simulink model "BenchmarkModel_Phasor"  (R2020a)
settings: Solver=VariableStepAuto  StartTime=0.0  StopTime=24*3600  RelTol=1e-3
undefined symbols (not defined in the file): A, a, Ac, B, Bc, C, Cc, Dc, Dd, find_system, Fnom, gcbh, I21_init_imag, I21_init_real, Ibase1, Ibase2, Iw1A_init_mag, Iw1A_init_pha, Iw1B_init_mag, Iw1B_init_pha, Iw1C_init_mag, Iw1C_init_pha, Iw2A_init_mag, Iw2A_init_pha, Iw2B_init_mag, Iw2B_init_pha, Iw2C_init_mag, Iw2C_init_pha, j, kr, ks, Nmax, Pnom, psi, sps_rtmsupport, V2G, Vnom1, Vnom2, w, Z1pu, Z2pu, Ztpu
libraries: powerlib x58, simulink x7, powerlib_meascontrol x7
(part 2 of 3)

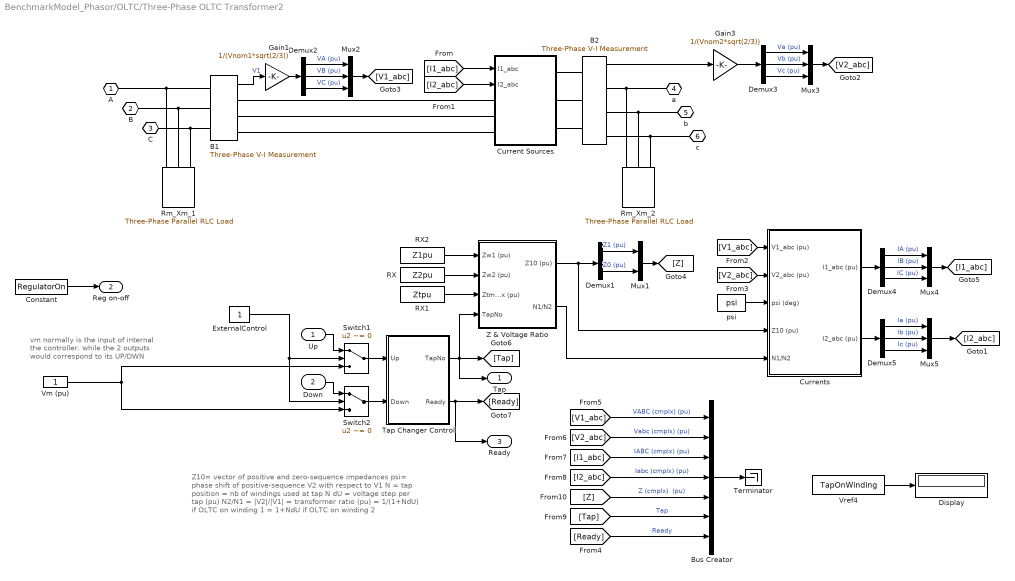
== system BenchmarkModel_Phasor/OLTC/Three-Phase OLTC Transformer2 ==
  note: vm normally is the input of
      | internal the controller.
      | while the 2 outputs would
      | correspond to its UP/DWN
  note: Z10= vector of positive and zero-sequence impedances
      | psi= phase shift of positive-sequence V2 with respect to V1
      | N =  tap position = nb of windings used at tap N
      | dU = voltage step  per tap (pu)
      | N2/N1 =  |V2|/|V1| = transformer ratio  (pu)
      |             = 1/(1+NdU)  if OLTC on winding 1
      |             = 1+NdU        if OLTC on winding 2
  Up : Inport
  Down : Inport  Port=2
  " Currents " : Subsystem
  "B1 " : powerlib/Measurements/Three-Phase V-I Measurement  VoltageMeasurement=phase-to-ground  SetLabelV=off  LabelV=Vabc_B21  Vpu=off  VpuLL=off  CurrentMeasurement=no  SetLabelI=off  LabelI=Iabc_B21  Ipu=off  Pbase=10e6  Vbase=Us  OutputType=Complex  PhasorSimulation=on  PSBequivalent=0
  B2 : powerlib/Measurements/Three-Phase V-I Measurement  VoltageMeasurement=phase-to-ground  SetLabelV=off  LabelV=Vabc_B21  Vpu=off  VpuLL=off  CurrentMeasurement=no  SetLabelI=off  LabelI=Iabc_B21  Ipu=off  Pbase=10e6  Vbase=Us  OutputType=Complex  PhasorSimulation=on  PSBequivalent=0
  Bus Creator : BusCreator  Inputs=7
  Constant : Constant  Value=RegulatorOn
  Current Sources : Subsystem
  Demux1 : Demux  Outputs=2
      settings: DisplayOption=none
  Demux{2..5} (4 alike) : Demux  Outputs=3
      settings: DisplayOption=none
  Display : Display
  ExternalControl : Constant
  Gain1 : Gain  Gain=1/(Vnom1*sqrt(2/3))  SaturateOnIntegerOverflow=on  OutDataTypeStr=Inherit: Same as input  ParamDataTypeStr=Inherit: Same as input
  Gain3 : Gain  Gain=1/(Vnom2*sqrt(2/3))  SaturateOnIntegerOverflow=on  OutDataTypeStr=Inherit: Same as input  ParamDataTypeStr=Inherit: Same as input
  Mux1 : Mux  Inputs=2
  Mux{2..5} (4 alike) : Mux  Inputs=3
  RX : Constant  Value=Z2pu
  RX1 : Constant  Value=Ztpu
  RX2 : Constant  Value=Z1pu
  Rm_Xm_1 : powerlib/Elements/Three-Phase Parallel RLC Load  LConnTagsString=A|B|C  Configuration=Y (grounded)  NominalVoltage=Vnom1  Vabc=[1e3 1e3 1e3]  Vabcp=[1e3 1e3 1e3]  NominalFrequency=Fnom  UnbalancedPower=off  ActivePower=Pnom/RmXm(1)/2  InductivePower=Pnom/RmXm(2)/2  CapacitivePower=0  Pabc=[10e3 9e3 11e3]  QLabc=[100 90 110]  QCabc=[100 90 110]  Pabcp=[10e3 9e3 11e3]  QLabcp=[100 90 110]  QCabcp=[100 90 110]  Measurements=None  LoadType=constant Z
  Rm_Xm_2 : powerlib/Elements/Three-Phase Parallel RLC Load  LConnTagsString=A|B|C  Configuration=Y (grounded)  NominalVoltage=Vnom2  Vabc=[1e3 1e3 1e3]  Vabcp=[1e3 1e3 1e3]  NominalFrequency=Fnom  UnbalancedPower=off  ActivePower=Pnom/RmXm(1)/2  InductivePower=Pnom/RmXm(2)/2  CapacitivePower=0  Pabc=[10e3 9e3 11e3]  QLabc=[100 90 110]  QCabc=[100 90 110]  Pabcp=[10e3 9e3 11e3]  QLabcp=[100 90 110]  QCabcp=[100 90 110]  Measurements=None  LoadType=constant Z
  Switch1 : Switch  Criteria=u2 ~= 0
  Switch2 : Switch  Criteria=u2 ~= 0
  Tap Changer Control : Subsystem  mask(Tap Changer Control){MinMaxTap=TapMinMax, InitialPosition=InitialTap, MecDelay=TapSelectionTime}
      mask prompts: MinMaxTap "Minimum and maximum tap number [ Min  Max ] :"; InitialPosition "Initial tap position"; MecDelay "Mechanical delay time"
      mask init:
      | if MecDelay<=0,
      | 	MecDelay=1/60;
      | end
  Terminator : Terminator
  Vm (pu) : Constant
  Vref4 : Constant  Value=TapOnWinding
  Z & Voltage Ratio : Subsystem
  psi : Constant  Value=psi
  A : PMIOPort  Tag=PMCPort  Side=Left
  B : PMIOPort  Tag=PMCPort  Port=2  Side=Left
  C : PMIOPort  Tag=PMCPort  Port=3  Side=Left
  a : PMIOPort  Tag=PMCPort  Port=4  Side=Right
  b : PMIOPort  Tag=PMCPort  Port=5  Side=Right
  c : PMIOPort  Tag=PMCPort  Port=6  Side=Right
  Tap : Outport
  Reg on-off : Outport  Port=2
  Ready : Outport  Port=3
  wires:
  [Ready] -> Bus Creator/7  "Ready"
  Constant/1 -> Reg on-off/1
  Switch2/1 -> Tap Changer Control/2("Down ")
  ExternalControl/1 -> Switch2/2, Switch1/2
  Down/1 -> Switch2/1
  Up/1 -> Switch1/1
  Switch1/1 -> Tap Changer Control/1("Up ")
  Vm (pu)/1 -> Switch2/3, Switch1/3
  Tap Changer Control/2(Ready) -> Ready/1, [Ready]
  Tap Changer Control/1(TapNo) -> Tap/1, Z & Voltage Ratio/4(TapNo), [Tap]
  "B1 "/1 -> Gain1/1  "V1"
  RX/1 -> Z & Voltage Ratio/2(Zw2 (pu))
  RX1/1 -> Z & Voltage Ratio/3(Ztmax (pu))
  Z & Voltage Ratio/1("Z10 (pu) ") -> Demux1/1, " Currents "/4(Z10 (pu))
  RX2/1 -> Z & Voltage Ratio/1(Zw1 (pu))
  Z & Voltage Ratio/2(N1/N2) -> " Currents "/5(N1/N2)
  [I1_abc] -> Current Sources/1(I1_abc)
  [I2_abc] -> Current Sources/2(I2_abc)
  B2/1 -> Gain3/1
  Gain3/1 -> Demux3/1
  Gain1/1 -> Demux2/1
  [V1_abc] -> " Currents "/1(V1_abc (pu))
  [V2_abc] -> " Currents "/2(V2_abc (pu))
  psi/1 -> " Currents "/3(psi (deg))
  [V2_abc] -> Bus Creator/2  "Vabc (cmplx) (pu)"
  Bus Creator/1 -> Terminator/1
  [I1_abc] -> Bus Creator/3  "IABC (cmplx) (pu)"
  [I2_abc] -> Bus Creator/4  "Iabc (cmplx) (pu)"
  [Tap] -> Bus Creator/6  "Tap"
  Demux1/1 -> Mux1/1  "Z1 (pu)"
  Demux1/2 -> Mux1/2  "Z0 (pu)"
  Mux1/1 -> [Z]
  [Z] -> Bus Creator/5  "Z (cmplx)  (pu)"
  Demux2/1 -> Mux2/1  "VA (pu)"
  Demux2/2 -> Mux2/2  "VB (pu)"
  Demux2/3 -> Mux2/3  "VC (pu)"
  Mux2/1 -> [V1_abc]
  [V1_abc] -> Bus Creator/1  "VABC (cmplx) (pu)"
  Demux3/1 -> Mux3/1  "Va (pu)"
  Demux3/2 -> Mux3/2  "Vb (pu)"
  Demux3/3 -> Mux3/3  "Vc (pu)"
  Mux3/1 -> [V2_abc]
  Demux4/1 -> Mux4/1  "IA (pu)"
  Demux4/2 -> Mux4/2  "IB (pu)"
  Demux4/3 -> Mux4/3  "IC (pu)"
  Mux4/1 -> [I1_abc]
  " Currents "/1(I1_abc (pu)) -> Demux4/1
  Demux5/1 -> Mux5/1  "Ia (pu)"
  Demux5/2 -> Mux5/2  "Ib (pu)"
  Demux5/3 -> Mux5/3  "Ic (pu)"
  Mux5/1 -> [I2_abc]
  " Currents "/2("I2_abc (pu) ") -> Demux5/1
  Vref4/1 -> Display/1
  connections:
  Current Sources/RConn3 -- B2/LConn3
  Current Sources/RConn2 -- B2/LConn2
  Current Sources/RConn1 -- B2/LConn1
  "B1 "/RConn3 -- Current Sources/LConn3
  "B1 "/RConn2 -- Current Sources/LConn2
  Current Sources/LConn1 -- "B1 "/RConn1
  A/RConn1 -- "B1 "/LConn1 -- Rm_Xm_1/LConn1
  B/RConn1 -- "B1 "/LConn2 -- Rm_Xm_1/LConn2
  C/RConn1 -- "B1 "/LConn3 -- Rm_Xm_1/LConn3
  c/RConn1 -- B2/RConn3 -- Rm_Xm_2/LConn3
  b/RConn1 -- B2/RConn2 -- Rm_Xm_2/LConn2
  a/RConn1 -- B2/RConn1 -- Rm_Xm_2/LConn1

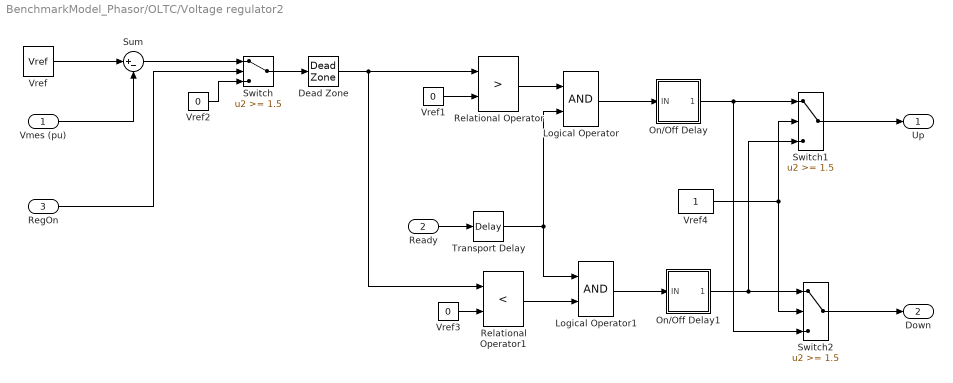
== system BenchmarkModel_Phasor/OLTC/Voltage regulator2 ==
  Vmes (pu) : Inport
  Ready : Inport  Port=2
  RegOn : Inport  Port=3
  Dead Zone : DeadZone  LowerValue=-DeadBand/2  UpperValue=+DeadBand/2  SaturateOnIntegerOverflow=on
  Logical Operator : Logic  AllPortsSameDT=off
  Logical Operator1 : Logic  AllPortsSameDT=off
  On/Off Delay : Subsystem  DialogController=POWERSYS.PowerSysDialog  mask(On/Off Delay){type_delay=On delay, delay=TimeDelay, ic=0}
      mask prompts: type_delay "Type:"; delay "Time delay:"; ic "Input at t = -eps (0/1):"
      mask help:
      | Apply a delay on the input signal when the input changes to TRUE (1) or FALSE (0).
      |
      | On delay: When the input becomes TRUE, the output becomes TRUE after the specified time delay as long as the input is still TRUE. If the input becomes FALSE before the time delay has expired , the output stays FALSE.
      |
      | Off delay: When the input becomes FALSE, the output becomes FALSE after the specified time delay as long as the input is still FALSE. If the input becomes TRUE before the time delay has expired , the output stays TRUE.
      |
      | The input value (0/1) at time preceding t=0 is specified by the parameter "input at t = -eps".
      mask init:
      | str=sprintf('%g %c',delay,'s');
      | power_initmask();
      mask Help: This block is part of a subset of blocks in the Extras library that does not have documentation associated with it, other than the block mask description.
      mask TypeOptions type_delay: On delay | Off delay
      mask Display:
      | plot(0,0,100,100,[10,10,10,90,90,90],[60,40,50,50,40,60]);
      | text(25+(type_delay-1)*50,80,'t');
      | text(15,20,str);
  On/Off Delay1 : Subsystem  DialogController=POWERSYS.PowerSysDialog  mask(On/Off Delay){type_delay=On delay, delay=TimeDelay, ic=0}
      mask prompts: type_delay "Type:"; delay "Time delay:"; ic "Input at t = -eps (0/1):"
      mask help:
      | Apply a delay on the input signal when the input changes to TRUE (1) or FALSE (0).
      |
      | On delay: When the input becomes TRUE, the output becomes TRUE after the specified time delay as long as the input is still TRUE. If the input becomes FALSE before the time delay has expired , the output stays FALSE.
      |
      | Off delay: When the input becomes FALSE, the output becomes FALSE after the specified time delay as long as the input is still FALSE. If the input becomes TRUE before the time delay has expired , the output stays TRUE.
      |
      | The input value (0/1) at time preceding t=0 is specified by the parameter "input at t = -eps".
      mask init:
      | str=sprintf('%g %c',delay,'s');
      | power_initmask();
      mask Help: This block is part of a subset of blocks in the Extras library that does not have documentation associated with it, other than the block mask description.
      mask TypeOptions type_delay: On delay | Off delay
      mask Display:
      | plot(0,0,100,100,[10,10,10,90,90,90],[60,40,50,50,40,60]);
      | text(25+(type_delay-1)*50,80,'t');
      | text(15,20,str);
  Relational Operator : RelationalOperator  Operator=>  RndMeth=Nearest
  Relational Operator1 : RelationalOperator  Operator=<  RndMeth=Nearest
  Sum : Sum  Inputs=|+-  SaturateOnIntegerOverflow=on
  Switch : Switch  Threshold=1.5  SaturateOnIntegerOverflow=on
  Switch1 : Switch  Threshold=1.5  SaturateOnIntegerOverflow=on
  Switch2 : Switch  Threshold=1.5  SaturateOnIntegerOverflow=on
  Transport Delay : TransportDelay  DelayTime=3/60  InitialOutput=1
  Vref : Constant  Value=Vref
  Vref1 : Constant  Value=0
  Vref2 : Constant  Value=0
  Vref3 : Constant  Value=0
  Vref4 : Constant
  "Up " : Outport
  "Down " : Outport  Port=2
  wires:
  Vref4/1 -> Switch2/2, Switch1/2
  Switch2/1 -> "Down "/1
  On/Off Delay1/1(OUT) -> Switch1/3, Switch2/1
  Switch1/1 -> "Up "/1
  On/Off Delay/1(OUT) -> Switch2/3, Switch1/1
  Vref2/1 -> Switch/3
  RegOn/1 -> Switch/2
  Switch/1 -> Dead Zone/1
  Sum/1 -> Switch/1
  Vref/1 -> Sum/1
  Vmes (pu)/1 -> Sum/2
  Dead Zone/1 -> Relational Operator1/1, Relational Operator/1
  Vref1/1 -> Relational Operator/2
  Relational Operator/1 -> Logical Operator/1
  Ready/1 -> Transport Delay/1
  Logical Operator/1 -> On/Off Delay/1(IN)
  Transport Delay/1 -> Logical Operator/2, Logical Operator1/1
  Vref3/1 -> Relational Operator1/2
  Relational Operator1/1 -> Logical Operator1/2
  Logical Operator1/1 -> On/Off Delay1/1(IN)

== system BenchmarkModel_Phasor/PV Farm/Avoid division by zero ==
  I : Inport
  Complex to Magnitude-Angle : ComplexToMagnitudeAngle
  Magnitude-Angle to Complex : MagnitudeAngleToComplex
  Saturation1 : Saturate  UpperLimit=inf  LowerLimit=1e-6
  O : Outport
  wires:
  Complex to Magnitude-Angle/2 -> Magnitude-Angle to Complex/2
  Magnitude-Angle to Complex/1 -> O/1
  Complex to Magnitude-Angle/1 -> Saturation1/1
  Saturation1/1 -> Magnitude-Angle to Complex/1
  I/1 -> Complex to Magnitude-Angle/1

== system BenchmarkModel_Phasor/PV Farm/Break Alg. Loop  ==
  In : Inport
  Complex to Real-Imag : ComplexToRealImag
  Real-Imag to Complex : RealImagToComplex
  imag : Subsystem  mask(Transfer Function with Initial Outputs){N=[1], D=[1  1], Y0=0, U0=0}
      mask prompts: N "Numerator:"; D "Denominator:"; Y0 "Initial output:"; U0 "Initial input:"
      mask help: Vector expressions for numerator, and denominator. Coefficients are in descending powers of s.
      mask init:
      | [A,B,C,Dd]=tf2ss(N,D);if (isempty(Y0));[m,n]=size(A);X0=zeros(1,m); end; if (isempty(U0));[m,p]=size(B);U0=zeros(1,p);end;X0=getxo(A,B,C,Dd,U0,Y0,0);
      mask Help: Specify the initial output for the transfer function.  An optimization routine attempts to determine the appropriate initial states so that the specified initial output is achieved.  For more details, see the m-file getxo.m
      mask Display: dpoly(N,D,'s')
  real : Subsystem  mask(Transfer Function with Initial Outputs){N=[1], D=[1  1], Y0=0, U0=0}
      mask prompts: N "Numerator:"; D "Denominator:"; Y0 "Initial output:"; U0 "Initial input:"
      mask help: Vector expressions for numerator, and denominator. Coefficients are in descending powers of s.
      mask init:
      | [A,B,C,Dd]=tf2ss(N,D);if (isempty(Y0));[m,n]=size(A);X0=zeros(1,m); end; if (isempty(U0));[m,p]=size(B);U0=zeros(1,p);end;X0=getxo(A,B,C,Dd,U0,Y0,0);
      mask Help: Specify the initial output for the transfer function.  An optimization routine attempts to determine the appropriate initial states so that the specified initial output is achieved.  For more details, see the m-file getxo.m
      mask Display: dpoly(N,D,'s')
  Out : Outport
  wires:
  imag/1(Out1) -> Real-Imag to Complex/2
  Complex to Real-Imag/2 -> imag/1(In1)
  real/1(Out1) -> Real-Imag to Complex/1
  Complex to Real-Imag/1 -> real/1(In1)
  Real-Imag to Complex/1 -> Out/1
  In/1 -> Complex to Real-Imag/1

== system BenchmarkModel_Phasor/PV Farm/Irradiance1 ==
  1-D Lookup IRRADIANCE Table : Lookup_n-D  NumberOfTableDimensions=1  BreakpointsForDimension1=V2G.IRRADIANCE.time  BeginIndexSearchUsingPreviousIndexResult=on  Table=V2G.IRRADIANCE.SUN  InternalRulePriority=Speed  RndMeth=Simplest  InputSameDT=on
  Add : Sum
  Clock1 : Clock
  Constant1 : Constant
  Second-->Hour : Gain  Gain=1/(60*60)
  " " : Outport
  wires:
  Constant1/1 -> Add/2
  Add/1 -> 1-D Lookup IRRADIANCE Table/1  "Hour of the day"
  1-D Lookup IRRADIANCE Table/1 -> " "/1
  Clock1/1 -> Second-->Hour/1
  Second-->Hour/1 -> Add/1

== system BenchmarkModel_Phasor/PV Farm/Partial Shading1 ==
  Add : Sum
  Clock : Clock
  Compare To Constant : simulink/Logic and Bit Operations/Compare To Constant  relop=>=  const=Ton  OutDataTypeStr=boolean
  Compare To Constant1 : simulink/Logic and Bit Operations/Compare To Constant  relop=<  const=Toff  OutDataTypeStr=boolean
  Constant : Constant  Value=Factor
  Logical Operator : Logic  AllPortsSameDT=off  OutDataTypeStr=float('double')
  Logical Operator1 : Logic  Operator=NOT  AllPortsSameDT=off  OutDataTypeStr=float('double')
  Product : Product
  Out : Outport
  wires:
  Add/1 -> Out/1
  Product/1 -> Add/2
  Constant/1 -> Product/2
  Compare To Constant/1 -> Logical Operator/1
  Clock/1 -> Compare To Constant1/1, Compare To Constant/1
  Compare To Constant1/1 -> Logical Operator/2
  Logical Operator/1 -> Logical Operator1/1, Product/1
  Logical Operator1/1 -> Add/1

== system BenchmarkModel_Phasor/Energy Storage System2/ESS Control/Charging Logic ==
  note: Charging is allowed between midnight and 6 o'clock in the morning if Stored Energy is less than 90 %
  Clk : Inport
  SE% : Inport  Port=2
  1 day in hours : Constant  Value=24
  Compare To Constant : simulink/Logic and Bit Operations/Compare To Constant  relop=<  const=Max  OutDataTypeStr=boolean
  Logical Operator1 : Logic  AllPortsSameDT=off  OutDataTypeStr=boolean
  Math Function : Math  Operator=mod  SignedPower=on  SaturateOnIntegerOverflow=on
  Scope{1..3,12} (4 alike) : Scope
  Second-->Hour : Gain  Gain=1/(60*60)
  night : simulink/Logic and Bit Operations/Compare To Constant  relop=<  const=6  OutDataTypeStr=boolean
  Charging On : Outport
  Night : Outport  Port=2
  wires:
  Logical Operator1/1 -> Scope1/1, Charging On/1
  Second-->Hour/1 -> Math Function/1
  Math Function/1 -> night/1
  1 day in hours/1 -> Math Function/2
  night/1 -> Night/1, Scope12/1, Logical Operator1/1
  SE%/1 -> Scope2/1, Compare To Constant/1
  Compare To Constant/1 -> Scope3/1, Logical Operator1/2
  Clk/1 -> Second-->Hour/1

== system BenchmarkModel_Phasor/Energy Storage System2/ESS Control/Regulator ==
  Reset : Inport
  On : Inport  Port=2
  Pmeas : Inport  Port=3
  Pref : Inport  Port=4
  Add1 : Sum  Inputs=|+-
  Integral Gain : Gain  Gain=Ki*1e3
  Integrator : Integrator  ExternalReset=falling  LimitOutput=on  UpperSaturationLimit=Plimit*1.1  LowerSaturationLimit=0
  Pref0 : Constant  Value=0
  Pref1 : Constant  Value=0
  Switch : Switch  Criteria=u2 ~= 0  Threshold=0.5
  Switch1 : Switch  Criteria=u2 ~= 0  Threshold=0.5
  Out : Outport
  tag scope: Error_pu=global
  wires:
  Reset/1 -> Integrator/2
  On/1 -> Switch1/2, Switch/2
  Pref0/1 -> Switch/3
  Pref1/1 -> Switch1/3
  Integral Gain/1 -> Integrator/1
  Switch/1 -> [Error_pu], Integral Gain/1
  Add1/1 -> Switch/1
  Integrator/1 -> Switch1/1
  Switch1/1 -> Out/1
  Pmeas/1 -> Add1/1
  Pref/1 -> Add1/2

== system BenchmarkModel_Phasor/Energy Storage System2/Inverter (Phasor)/Avoid division by zero ==
  I : Inport
  Complex to Magnitude-Angle : ComplexToMagnitudeAngle
  Magnitude-Angle to Complex : MagnitudeAngleToComplex
  Saturation1 : Saturate  UpperLimit=inf  LowerLimit=1e-6
  O : Outport
  wires:
  I/1 -> Complex to Magnitude-Angle/1
  Saturation1/1 -> Magnitude-Angle to Complex/1
  Complex to Magnitude-Angle/1 -> Saturation1/1
  Magnitude-Angle to Complex/1 -> O/1
  Complex to Magnitude-Angle/2 -> Magnitude-Angle to Complex/2

== system BenchmarkModel_Phasor/Energy Storage System2/Inverter (Phasor)/Break Alg. Loop  ==
  In : Inport
  Complex to Real-Imag : ComplexToRealImag
  Real-Imag to Complex : RealImagToComplex
  imag : Subsystem  mask(Transfer Function with Initial Outputs){N=[1], D=[1  1], Y0=0, U0=0}
      mask prompts: N "Numerator:"; D "Denominator:"; Y0 "Initial output:"; U0 "Initial input:"
      mask help: Vector expressions for numerator, and denominator. Coefficients are in descending powers of s.
      mask init:
      | [A,B,C,Dd]=tf2ss(N,D);if (isempty(Y0));[m,n]=size(A);X0=zeros(1,m); end; if (isempty(U0));[m,p]=size(B);U0=zeros(1,p);end;X0=getxo(A,B,C,Dd,U0,Y0,0);
      mask Help: Specify the initial output for the transfer function.  An optimization routine attempts to determine the appropriate initial states so that the specified initial output is achieved.  For more details, see the m-file getxo.m
      mask Display: dpoly(N,D,'s')
  real : Subsystem  mask(Transfer Function with Initial Outputs){N=[1], D=[1  1], Y0=0, U0=0}
      mask prompts: N "Numerator:"; D "Denominator:"; Y0 "Initial output:"; U0 "Initial input:"
      mask help: Vector expressions for numerator, and denominator. Coefficients are in descending powers of s.
      mask init:
      | [A,B,C,Dd]=tf2ss(N,D);if (isempty(Y0));[m,n]=size(A);X0=zeros(1,m); end; if (isempty(U0));[m,p]=size(B);U0=zeros(1,p);end;X0=getxo(A,B,C,Dd,U0,Y0,0);
      mask Help: Specify the initial output for the transfer function.  An optimization routine attempts to determine the appropriate initial states so that the specified initial output is achieved.  For more details, see the m-file getxo.m
      mask Display: dpoly(N,D,'s')
  Out : Outport
  wires:
  In/1 -> Complex to Real-Imag/1
  Real-Imag to Complex/1 -> Out/1
  Complex to Real-Imag/1 -> real/1(In1)
  real/1(Out1) -> Real-Imag to Complex/1
  Complex to Real-Imag/2 -> imag/1(In1)
  imag/1(Out1) -> Real-Imag to Complex/2

== system BenchmarkModel_Phasor/Load Residential = 30 kW, PF=0.95/Residential Load1/Avoid division by zero ==
  I : Inport
  Complex to Magnitude-Angle : ComplexToMagnitudeAngle
  Magnitude-Angle to Complex : MagnitudeAngleToComplex
  Saturation1 : Saturate  UpperLimit=inf  LowerLimit=1e-6
  O : Outport  VectorParamsAs1DForOutWhenUnconnected=off
  wires:
  I/1 -> Complex to Magnitude-Angle/1
  Saturation1/1 -> Magnitude-Angle to Complex/1
  Complex to Magnitude-Angle/1 -> Saturation1/1
  Magnitude-Angle to Complex/1 -> O/1
  Complex to Magnitude-Angle/2 -> Magnitude-Angle to Complex/2

== system BenchmarkModel_Phasor/Load Residential = 30 kW, PF=0.95/Residential Load1/Break Alg. Loop 1 ==
  In : Inport
  Complex to Real-Imag : ComplexToRealImag
  Real-Imag to Complex : RealImagToComplex
  imag1 : Subsystem  mask(Transfer Function with Initial Outputs){N=[1], D=[1  1], Y0=0, U0=0}
      mask prompts: N "Numerator:"; D "Denominator:"; Y0 "Initial output:"; U0 "Initial input:"
      mask help: Vector expressions for numerator, and denominator. Coefficients are in descending powers of s.
      mask init:
      | [A,B,C,Dd]=tf2ss(N,D);if (isempty(Y0));[m,n]=size(A);X0=zeros(1,m); end; if (isempty(U0));[m,p]=size(B);U0=zeros(1,p);end;X0=getxo(A,B,C,Dd,U0,Y0,0);
      mask Help: Specify the initial output for the transfer function.  An optimization routine attempts to determine the appropriate initial states so that the specified initial output is achieved.  For more details, see the m-file getxo.m
      mask Display: dpoly(N,D,'s')
  real1 : Subsystem  mask(Transfer Function with Initial Outputs){N=[1], D=[1  1], Y0=0, U0=0}
      mask prompts: N "Numerator:"; D "Denominator:"; Y0 "Initial output:"; U0 "Initial input:"
      mask help: Vector expressions for numerator, and denominator. Coefficients are in descending powers of s.
      mask init:
      | [A,B,C,Dd]=tf2ss(N,D);if (isempty(Y0));[m,n]=size(A);X0=zeros(1,m); end; if (isempty(U0));[m,p]=size(B);U0=zeros(1,p);end;X0=getxo(A,B,C,Dd,U0,Y0,0);
      mask Help: Specify the initial output for the transfer function.  An optimization routine attempts to determine the appropriate initial states so that the specified initial output is achieved.  For more details, see the m-file getxo.m
      mask Display: dpoly(N,D,'s')
  Out : Outport  VectorParamsAs1DForOutWhenUnconnected=off
  wires:
  In/1 -> Complex to Real-Imag/1
  Real-Imag to Complex/1 -> Out/1
  real1/1(Out1) -> Real-Imag to Complex/1
  Complex to Real-Imag/1 -> real1/1(In1)
  imag1/1(Out1) -> Real-Imag to Complex/2
  Complex to Real-Imag/2 -> imag1/1(In1)

== system BenchmarkModel_Phasor/Load Residential = 30 kW, PF=0.95/Residential Load1/Load_profile ==
  Add : Sum
  Clock : Clock
  Constant : Constant
  Constant1 : Constant  Value=PF
  Divide : Product  Inputs=*/
  Mux : Mux  Inputs=2
  P nom : Constant  Value=-nomPower*1e3
  Power consumption : Lookup_n-D  NumberOfTableDimensions=1  BreakpointsForDimension1=[timestep/60:timestep/60:24]  BeginIndexSearchUsingPreviousIndexResult=on  Table=|  InternalRulePriority=Speed  RndMeth=Simplest  InputSameDT=on
      | [0.677944961393784
      | 0.642981587804395
      | 0.671609582260939
      | 0.643694317956840
      | 0.648723025143536
      | 0.582993466640269
      | 0.552860819639675
      | 0.559730746386854
      | 0.505147495545437
      | 0.539239754504059
      | 0.541160166303702
      | 0.520431597703425
      | 0.491922391605623
      | 0.456345278162740
      | 0.434409027915264
      | 0.407840031676896
      | 0.379588200356365
      | 0.345792912294595
      | 0.346208671550188
      | 0.350188081568006
      | 0.353652742031281
      | 0.335735497921204
      | 0.327598495347456
      | 0.334646604632746
      | 0.340190061373985
      | 0.364561472975648
      | 0.352484656503663
      | 0.357275786972877
      | 0.358047911304692
      | 0.376163136012671
      | 0.373747772718274
      | 0.386299742625223
      | 0.395426648188478
      | 0.408077608394377
      | 0.456840229657494
      | 0.494278360720649
      | 0.489012076816472
      | 0.508117204513958
      | 0.583963571569986
      | 0.629083349831717
      | 0.601128489408038
      | 0.661195802811325
      | 0.663670560285092
      | 0.703207285686003
      | 0.802771728370620
      | 0.793486438329044
      | 0.859889130865175
      | 0.980696891704613
      | 0.959592159968323
      | 0.997782617303504
      | 0.972500494951495
      | 0.952900415759256
      | 0.900356365076223
      | 0.823539893090477
      | 0.822490595921600
      | 0.807998416155217
      | 0.776539299148683
      | 0.694139774302118
      | 0.673193427044150
      | 0.657612353989309
      | 0.685963175608790
      | 0.723836863987329
      | 0.785804791130469
      | 0.738606216590774
      | 0.757176796673926
      | 0.722272817263908
      | 0.795624628786379
      | 0.847020392001584
      | 0.914393189467432
      | 0.892892496535339
      | 0.895010888932885
      | 0.874420906751138
      | 0.915640467234211
      | 0.946802613343892
      | 0.977133240942388
      | 0.962502474757474
      | 0.970758265689962
      | 0.996931300732528
      | 0.978103345872105
      | 1
      | 0.993031082953870
      | 0.987091665016828
      | 0.960205899821817
      | 0.985804791130469
      | 0.904672342110473
      | 0.866897644030885
      | 0.846050287071867
      | 0.836982775687983
      | 0.852405464264502
      | 0.830013858641853
      | 0.791308651752128
      | 0.756939219956444
      | 0.765590972084736
      | 0.731934270441497
      | 0.675846367056029
      | 0.678321124529796]
  Product : Product
  Product1 : Product
  Second-->Hour : Gain  Gain=1/(60*60)
  Trigonometric Function : Trigonometry
  Trigonometric Function1 : Trigonometry  Operator=acos
  PQ : Outport
  wires:
  Constant/1 -> Add/2
  Second-->Hour/1 -> Add/1
  Add/1 -> Power consumption/1
  P nom/1 -> Product/2
  Clock/1 -> Second-->Hour/1
  Product/1 -> Divide/1, Mux/1
  Power consumption/1 -> Product/1
  Mux/1 -> PQ/1
  Trigonometric Function1/1 -> Trigonometric Function/1
  Constant1/1 -> Divide/2, Trigonometric Function1/1
  Trigonometric Function/1 -> Product1/2
  Divide/1 -> Product1/1
  Product1/1 -> Mux/2

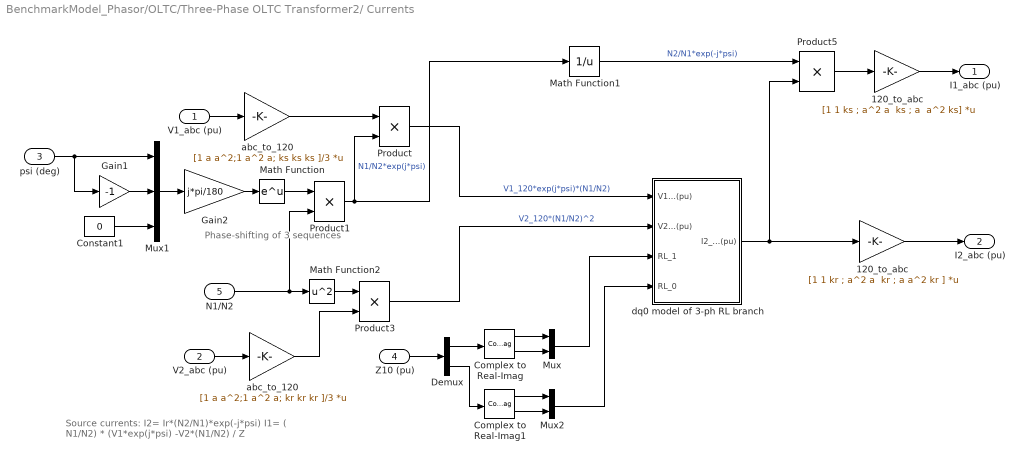
== system BenchmarkModel_Phasor/OLTC/Three-Phase OLTC Transformer2/ Currents  ==
  note: Phase-shifting
      | of 3 sequences
  note: Source currents:
      |
      | I2= Ir*(N2/N1)*exp(-j*psi)
      | I1= ( N1/N2) * (V1*exp(j*psi) -V2*(N1/N2) / Z
  V1_abc (pu) : Inport
  V2_abc (pu) : Inport  Port=2
  psi (deg) : Inport  Port=3
  Z10 (pu) : Inport  Port=4
  N1/N2 : Inport  Port=5
  120_to_abc : Gain  Gain="[1 1 kr ; a^2 a  kr ; a a^2 kr ]"  Multiplication=Matrix(K*u)  SaturateOnIntegerOverflow=on  OutDataTypeStr=Inherit: Same as input  ParamDataTypeStr=Inherit: Same as input
  "120_to_abc " : Gain  Gain="[1 1 ks ; a^2 a  ks ; a  a^2 ks]"  Multiplication=Matrix(K*u)  SaturateOnIntegerOverflow=on  OutDataTypeStr=Inherit: Same as input  ParamDataTypeStr=Inherit: Same as input
  Complex to Real-Imag : ComplexToRealImag
  Complex to Real-Imag1 : ComplexToRealImag
  Constant1 : Constant  Value=0
  Demux : Demux  Outputs=2
      settings: DisplayOption=none
  Gain1 : Gain  Gain=-1  SaturateOnIntegerOverflow=on  OutDataTypeStr=Inherit: Same as input  ParamDataTypeStr=Inherit: Same as input
  Gain2 : Gain  Gain=j*pi/180  SaturateOnIntegerOverflow=on  OutDataTypeStr=Inherit: Same as input  ParamDataTypeStr=Inherit: Same as input
  Math Function : Math  SignedPower=on  SaturateOnIntegerOverflow=on
  Math Function1 : Math  Operator=reciprocal  SignedPower=on  SaturateOnIntegerOverflow=on
  Math Function2 : Math  Operator=square  SignedPower=on  SaturateOnIntegerOverflow=on
  Mux : Mux  Inputs=2
  Mux1 : Mux  Inputs=3
  Mux2 : Mux  Inputs=2
  Product : Product  SaturateOnIntegerOverflow=on  OutDataTypeStr=Inherit: Same as first input
  Product1 : Product  Inputs=**  SaturateOnIntegerOverflow=on  OutDataTypeStr=Inherit: Same as first input
  Product3 : Product  Inputs=**  SaturateOnIntegerOverflow=on  OutDataTypeStr=Inherit: Same as first input
  Product5 : Product  SaturateOnIntegerOverflow=on  OutDataTypeStr=Inherit: Same as first input
  abc_to_120 : Gain  Gain=[1 a a^2;1 a^2 a; ks ks ks ]/3  Multiplication=Matrix(K*u)  SaturateOnIntegerOverflow=on  OutDataTypeStr=Inherit: Same as input  ParamDataTypeStr=Inherit: Same as input
  "abc_to_120 " : Gain  Gain=[1 a a^2;1 a^2 a; kr kr kr ]/3  Multiplication=Matrix(K*u)  SaturateOnIntegerOverflow=on  OutDataTypeStr=Inherit: Same as input  ParamDataTypeStr=Inherit: Same as input
  dq0 model of 3-ph RL branch : Subsystem
  I1_abc (pu) : Outport
  "I2_abc (pu) " : Outport  Port=2
  wires:
  Gain2/1 -> Math Function/1
  Product/1 -> dq0 model of 3-ph RL branch/1(V1_120(pu))  "V1_120*exp(j*psi)*(N1/N2)"
  Product3/1 -> dq0 model of 3-ph RL branch/2(V2_120(pu))  "V2_120*(N1/N2)^2"
  N1/N2/1 -> Product1/2, Math Function2/1
  Product1/1 -> Math Function1/1, Product/2  "N1/N2*exp(j*psi)"
  Math Function/1 -> Product1/1
  V1_abc (pu)/1 -> abc_to_120/1
  V2_abc (pu)/1 -> "abc_to_120 "/1
  Product5/1 -> "120_to_abc "/1
  abc_to_120/1 -> Product/1
  Math Function1/1 -> Product5/1  "N2/N1*exp(-j*psi)"
  psi (deg)/1 -> Gain1/1, Mux1/1
  Mux1/1 -> Gain2/1
  Gain1/1 -> Mux1/2
  Constant1/1 -> Mux1/3
  "abc_to_120 "/1 -> Product3/2
  120_to_abc/1 -> "I2_abc (pu) "/1
  "120_to_abc "/1 -> I1_abc (pu)/1
  Z10 (pu)/1 -> Demux/1
  Demux/1 -> Complex to Real-Imag/1
  Demux/2 -> Complex to Real-Imag1/1
  Complex to Real-Imag/1 -> Mux/1
  Complex to Real-Imag/2 -> Mux/2
  Mux/1 -> dq0 model of 3-ph RL branch/3(RL_1)
  Complex to Real-Imag1/1 -> Mux2/1
  Complex to Real-Imag1/2 -> Mux2/2
  Mux2/1 -> dq0 model of 3-ph RL branch/4(RL_0)
  dq0 model of 3-ph RL branch/1(I2_120 (pu)) -> 120_to_abc/1, Product5/2
  Math Function2/1 -> Product3/1

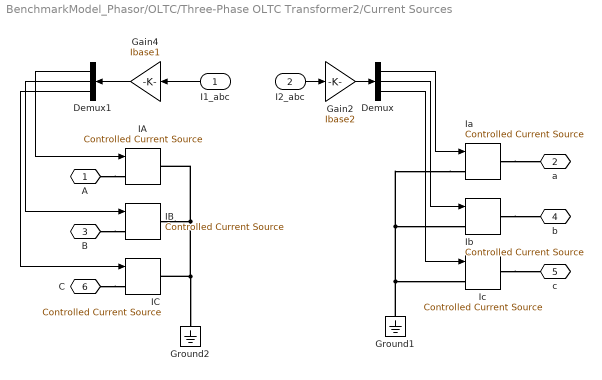
== system BenchmarkModel_Phasor/OLTC/Three-Phase OLTC Transformer2/Current Sources ==
  I1_abc : Inport
  I2_abc : Inport  Port=2
  Demux : Demux  Outputs=3
      settings: DisplayOption=none
  Demux1 : Demux  Outputs=3
      settings: DisplayOption=none
  Gain2 : Gain  Gain=Ibase2  SaturateOnIntegerOverflow=on  OutDataTypeStr=Inherit: Same as input  ParamDataTypeStr=Inherit: Same as input
  Gain4 : Gain  Gain=Ibase1  SaturateOnIntegerOverflow=on  OutDataTypeStr=Inherit: Same as input  ParamDataTypeStr=Inherit: Same as input
  Ground1 : powerlib/Elements/Ground  LConnTagsString=a
  Ground2 : powerlib/Elements/Ground  LConnTagsString=a
  IA : powerlib/Electrical Sources/Controlled Current Source  Initialize=on  Source_Type=AC  Amplitude=Iw1A_init_mag  Phase=Iw1A_init_pha  Frequency=Fnom  Measurements=None
  IB : powerlib/Electrical Sources/Controlled Current Source  Initialize=on  Source_Type=AC  Amplitude=Iw1B_init_mag  Phase=Iw1B_init_pha  Frequency=Fnom  Measurements=None
  IC : powerlib/Electrical Sources/Controlled Current Source  Initialize=on  Source_Type=AC  Amplitude=Iw1C_init_mag  Phase=Iw1C_init_pha  Frequency=Fnom  Measurements=None
  Ia : powerlib/Electrical Sources/Controlled Current Source  Initialize=on  Source_Type=AC  Amplitude=Iw2A_init_mag  Phase=Iw2A_init_pha  Frequency=Fnom  Measurements=None
  Ib : powerlib/Electrical Sources/Controlled Current Source  Initialize=on  Source_Type=AC  Amplitude=Iw2B_init_mag  Phase=Iw2B_init_pha  Frequency=Fnom  Measurements=None
  Ic : powerlib/Electrical Sources/Controlled Current Source  Initialize=on  Source_Type=AC  Amplitude=Iw2C_init_mag  Phase=Iw2C_init_pha  Frequency=Fnom  Measurements=None
  A : PMIOPort  Side=Left
  a : PMIOPort  Port=2  Side=Right
  B : PMIOPort  Port=3  Side=Left
  b : PMIOPort  Port=4  Side=Right
  c : PMIOPort  Port=5  Side=Right
  C : PMIOPort  Port=6  Side=Left
  wires:
  I1_abc/1 -> Gain4/1
  I2_abc/1 -> Gain2/1
  Demux/3 -> Ic/1
  Demux/2 -> Ib/1
  Demux/1 -> Ia/1
  Demux1/3 -> IC/1
  Demux1/2 -> IB/1
  Demux1/1 -> IA/1
  Gain2/1 -> Demux/1
  Gain4/1 -> Demux1/1
  connections:
  Ic/RConn1 -- c/RConn1
  Ib/RConn1 -- b/RConn1
  Ia/RConn1 -- a/RConn1
  C/RConn1 -- IC/LConn1
  B/RConn1 -- IB/LConn1
  A/RConn1 -- IA/LConn1
  Ia/LConn1 -- Ib/LConn1 -- Ic/LConn1 -- Ground1/LConn1
  IB/RConn1 -- IA/RConn1 -- IC/RConn1 -- Ground2/LConn1

== system BenchmarkModel_Phasor/OLTC/Three-Phase OLTC Transformer2/Tap Changer Control ==
  "Up " : Inport
  "Down " : Inport  Port=2
  Constant : Constant  Value=-1
  Constant1 : Constant
  Determine tap position : Subsystem
  Edge Detector : Subsystem  DialogController=POWERSYS.PowerSysDialog  mask(Edge Detector){model=Rising, ic=0}
      mask prompts: model "Edge:"; ic "Input at t = -eps:"
      mask help:
      | This block compares its present input to its previous input.
      |
      | If the input  is a logic signal (TRUE (1) or FALSE (0), the output is a one-step boolean signal TRUE  when  the specified edge (Rising, Falling or Either)  is detected.
      |
      | This block can also be used to detect the slope polarity of a continuous signal. For example, if the specified edge is  "Rising", the output is TRUE as long as the slope of the input signal is positive.
      |
      | The input value at time preceding t=0 is specified by the parameter "Input at t=-eps"
      mask init:
      | if model~=3,
      | 	x1 = (model -1)*20;
      |     x2 = (model -1)*60;
      | 	X1=[5,20,20,35]+25; Y1=[20+x2,20+x2,80-x2,80-x2];
      | 	X2=[5,20,35]+25;    Y2=[40+x1,60-x1,40+x1];
      | 	X3=[];X4=[];Y3=[];Y4=[];
      | else
      | 	x1 = 20;
      | 	x2 = 60;
      | 	X1=[5,20,20,35]+8; Y1=[20,20,80,80];
      | 	X2=[5,20,35]+8;    Y2=[40,60,40];
      | 	X3=[5,20,20,35]+53; Y3=[20+x2,20+x2,80-x2,80-x2];
      | 	X4=[5,20,35]+53;    Y4=[40+x1,60-x1,40+x1];
      | end
      | power_initmask();
      mask Help: This block is part of a subset of blocks in the Extras library that does not have documentation associated with it, other than the block mask description.
      mask TypeOptions model: Rising | Falling | Either
      mask Display: plot(0,0,100,100, X1,Y1,X2,Y2,X3,Y3,X4,Y4);
  Logical Operator : Logic  Operator=OR  AllPortsSameDT=off
  Logical Operator1 : Logic  AllPortsSameDT=off
  Mechanical Delay : TransportDelay  DelayTime=MecDelay  InitialOutput=InitialPosition
  Memory : Memory  InitialCondition=1  InheritSampleTime=on
  Relational Operator : RelationalOperator  Operator===  OutDataTypeStr=float('double')  RndMeth=Nearest
  Switch : Switch  Threshold=0.5  SaturateOnIntegerOverflow=on
  TapNo : Outport
  Ready : Outport  Port=2
  wires:
  Edge Detector/1(Out) -> Logical Operator1/2
  Logical Operator/1 -> Edge Detector/1(In)
  Memory/1 -> Ready/1, Logical Operator1/1
  Relational Operator/1 -> Memory/1
  Determine tap position/1(TapNo) -> Relational Operator/1, Mechanical Delay/1
  Switch/1 -> Determine tap position/1(NewTap)
  Constant1/1 -> Switch/3
  Constant/1 -> Switch/1
  "Down "/1 -> Switch/2, Logical Operator/2
  "Up "/1 -> Logical Operator/1
  Logical Operator1/1 -> Determine tap position/Trigger
  Mechanical Delay/1 -> Relational Operator/2, TapNo/1

== system BenchmarkModel_Phasor/OLTC/Three-Phase OLTC Transformer2/Z & Voltage Ratio ==
  note: Z10= vector of positive and zero-sequence impedances
      | psi= phase shift of  V2 with respect to V1 for positive-sequence
      | N2/N1 =  |V2|/|V1| = transformer ratio
      | N = nb of windings used at tap N
      | dU = voltage step  per tap (pu)
  Zw1 (pu) : Inport
  Zw2 (pu) : Inport  Port=2
  Ztmax (pu) : Inport  Port=3
  TapNo : Inport  Port=4
  1st-Order Filter4 : Subsystem  DialogController=POWERSYS.PowerSysDialog  mask(First-Order Filter){FilterType=Lowpass, Tc=1/Fnom, Initialize=on, Vac_Init=[0 0  Fnom], Vdc_Init=InitialTap, PlotResponse=off, param1=[1 500 1]}
      mask prompts: FilterType "Filter Type:"; Tc "Time constant (s):"; Initialize "Initialize filter states"; Vac_Init "AC initial input: [ Mag  Phase(degrees)  Freq(Hz) ]"; Vdc_Init "DC Initial input:"; PlotResponse "Plot filter response"; param1 "Frequency range(Hz) : [Start  End  Inc.]"
      mask init:
      | switch FilterType
      | case 1, % Lowpass
      |        X=[0 1 2 3 4];
      |        Y=[-2 -2 -3 -4 -4];
      |        numc=1;
      |        denc=[Tc 1];
      |  case 2,   % Highpass
      |        X=[0 1 2 3 4];
      |        Y=[-4 -4 -3 -2 -2];
      |         numc=[1 0];
      |         denc=[1 1/Tc];
      | end
      | %
      | [Ac,Bc,Cc,Dc]=tf2ss(numc,denc);
      | %
      | %
      | if Initialize==1  % Compute initial conditions on states
      | u1=Vac_Init(1)*exp(j*Vac_Init(2)*pi/180);
      | u2=Vdc_Init*exp(j*90*pi/180);
      | u=u1+u2;
      | u0=imag(u); % input at  t=0;
      | I=eye(size(Ac));
      | sI1=I*j*(2*pi*Vac_Init(3));
      | sI2=I*j*0;
      | x=inv(sI1-Ac)*Bc*u1 + inv(sI2-Ac)*Bc*u2;
      | x0c=imag(x);
      | else
      | x0c=0;
      | end
      | %
      | if PlotResponse==1 % Plot frequency and step response
      | t=[0:Tc/1000:7*Tc];
      | f=param1(1):param1(3):param1(2);
      | w=2*pi*f;
      | switch FilterType
      | 	case 1, % Lowpass
      | 		Ystep=1 - exp(-t/Tc);
      | 		RepFreq=1./(1+Tc*j.*w);
      | 	case 2,   % Highpass
      | 		Ystep=exp(-t/Tc);
      | 		RepFreq=1./(1 + (1./(Tc*j.*w)));
      | end
      | %
      | Mag=abs(RepFreq);
      | Pha=angle(RepFreq)*180/pi;
      | %
      | figure(1)
      | subplot(2,1,1)
      | plot(f,Mag)
      | grid
      | title('Bode Diagram')
      | ylabel('Magnitude')
      | subplot(2,1,2)
      | plot(f,Pha)
      | ylabel('Phase (deg)')
      | xlabel('Frequency (Hz)')
      | grid
      | figure(2)
      | plot(t,Ystep)
      | grid
      | ylabel('Amplitude')
      | xlabel('Time (s)')
      | title('Step Response')
      | end
      | power_initmask();
      mask Help: This block is part of a subset of blocks in the Extras library that does not have documentation associated with it, other than the block mask description.
      mask TypeOptions FilterType: Lowpass | Highpass
      mask Callback Initialize: %parametres=get_param(gcb,'MaskValues');p3=parametres{3};p6=parametres{6};if strcmp(p3,'on');param4='on';param5='on';else;param4='off';param5='off';end;if strcmp(p6,'on');param7='on';else;param7='off';end;visible={'on','on','on',param4,param5,'on',param7};set_param(gcb,'MaskVisibilities',visible)
      mask Callback PlotResponse: %parametres=get_param(gcb,'MaskValues');p3=parametres{3};p6=parametres{6};if strcmp(p3,'on');param4='on';param5='on';else;param4='off';param5='off';end;if strcmp(p6,'on');param7='on';else;param7='off';end;visible={'on','on','on',param4,param5,'on',param7};set_param(gcb,'MaskVisibilities',visible)
      mask Display: plot(X,Y);
  Logical Operator : Logic  Operator=NOT  AllPortsSameDT=off
  Mux : Mux  Inputs=2
  RX1 : Constant  Value=TapOnWinding
  RX2 : Constant
  RX3 : Constant  Value=dU
  RX4 : Constant  Value=Nmax
  Relational Operator : RelationalOperator  Operator===  RndMeth=Nearest
  Switch : Switch  Criteria=u2 ~= 0  Threshold=0.5  SaturateOnIntegerOverflow=on
  Switch1 : Switch  Criteria=u2 ~= 0  Threshold=0.5  SaturateOnIntegerOverflow=on
  Z Tap on winding 1 : Subsystem
  Z Tap on winding 2 : Subsystem
  "Z10 (pu) " : Outport
  N1/N2 : Outport  Port=2
  wires:
  RX4/1 -> Z Tap on winding 2/6(Nmax), Z Tap on winding 1/6(Nmax)
  TapNo/1 -> 1st-Order Filter4/1(In)  "N"
  1st-Order Filter4/1(Out) -> Z Tap on winding 1/1(N), Z Tap on winding 2/1(N)  "N"
  Zw2 (pu)/1 -> Z Tap on winding 1/4(Zw2), Z Tap on winding 2/4(Zw2)
  Zw1 (pu)/1 -> Z Tap on winding 1/3(Zw1), Z Tap on winding 2/3(Zw1)
  RX1/1 -> Relational Operator/1
  RX2/1 -> Relational Operator/2
  Relational Operator/1 -> Z Tap on winding 1/Enable, Logical Operator/1, Switch/2, Switch1/2
  Logical Operator/1 -> Z Tap on winding 2/Enable
  Z Tap on winding 1/1(Z) -> Switch/1
  Z Tap on winding 2/1(Z) -> Switch/3
  Z Tap on winding 1/2(N1/N2) -> Switch1/1
  Z Tap on winding 2/2(N1/N2) -> Switch1/3
  Switch1/1 -> N1/N2/1
  Ztmax (pu)/1 -> Z Tap on winding 1/5(Ztmax), Z Tap on winding 2/5(Ztmax)
  RX3/1 -> Z Tap on winding 1/2(dU), Z Tap on winding 2/2(dU)
  Switch/1 -> Mux/1, Mux/2
  Mux/1 -> "Z10 (pu) "/1

== system BenchmarkModel_Phasor/OLTC/Voltage regulator2/On//Off Delay ==
  note: Silvano Casoria
      | Power System Simulation Laboratory
      | IREQ, Hydro-Quebc
  note: On/Off Delay
  IN : Inport
  Clock : Clock
  Constant : Constant
  Constant1 : Constant  Value=delay
  Constant2 : Constant  Value=type_delay
  Data Type Conversion1 : DataTypeConversion  OutDataTypeStr=boolean  SaturateOnIntegerOverflow=on  RndMeth=Zero
  Logical Operator1 : Logic  Operator=OR
  Logical Operator2 : Logic  Operator=NOT  Inputs=1
  OFF Delay : Subsystem  TreatAsAtomicUnit=on
  ON Delay : Subsystem  TreatAsAtomicUnit=on
  Relational Operator1 : RelationalOperator  Operator===  RndMeth=Nearest  InputSameDT=on
  OUT : Outport
  wires:
  Data Type Conversion1/1 -> OFF Delay/1(IN), ON Delay/1(IN)
  Constant/1 -> Relational Operator1/2
  Relational Operator1/1 -> ON Delay/Enable, Logical Operator2/1
  Constant2/1 -> Relational Operator1/1
  Logical Operator2/1 -> OFF Delay/Enable
  OFF Delay/1(OUT) -> Logical Operator1/2
  ON Delay/1(OUT) -> Logical Operator1/1
  Logical Operator1/1 -> OUT/1
  Constant1/1 -> ON Delay/3(DELAY), OFF Delay/3(DELAY)
  IN/1 -> Data Type Conversion1/1
  Clock/1 -> OFF Delay/2(clock), ON Delay/2(clock)

== system BenchmarkModel_Phasor/OLTC/Voltage regulator2/On//Off Delay1 ==
  note: Silvano Casoria
      | Power System Simulation Laboratory
      | IREQ, Hydro-Quebc
  note: On/Off Delay
  IN : Inport
  Clock : Clock
  Constant : Constant
  Constant1 : Constant  Value=delay
  Constant2 : Constant  Value=type_delay
  Data Type Conversion1 : DataTypeConversion  OutDataTypeStr=boolean  SaturateOnIntegerOverflow=on  RndMeth=Zero
  Logical Operator1 : Logic  Operator=OR
  Logical Operator2 : Logic  Operator=NOT  Inputs=1
  OFF Delay : Subsystem  TreatAsAtomicUnit=on
  ON Delay : Subsystem  TreatAsAtomicUnit=on
  Relational Operator1 : RelationalOperator  Operator===  RndMeth=Nearest  InputSameDT=on
  OUT : Outport
  wires:
  Data Type Conversion1/1 -> OFF Delay/1(IN), ON Delay/1(IN)
  Constant/1 -> Relational Operator1/2
  Relational Operator1/1 -> ON Delay/Enable, Logical Operator2/1
  Constant2/1 -> Relational Operator1/1
  Logical Operator2/1 -> OFF Delay/Enable
  OFF Delay/1(OUT) -> Logical Operator1/2
  ON Delay/1(OUT) -> Logical Operator1/1
  Logical Operator1/1 -> OUT/1
  Constant1/1 -> ON Delay/3(DELAY), OFF Delay/3(DELAY)
  IN/1 -> Data Type Conversion1/1
  Clock/1 -> OFF Delay/2(clock), ON Delay/2(clock)

== system BenchmarkModel_Phasor/PV Farm/Break Alg. Loop /imag ==
  In1 : Inport
  State Space : StateSpace  A=A  B=B  C=C  D=Dd  InitialCondition=X0
  Out1 : Outport  InitialOutput=0
  wires:
  In1/1 -> State Space/1
  State Space/1 -> Out1/1

== system BenchmarkModel_Phasor/PV Farm/Break Alg. Loop /real ==
  In1 : Inport
  State Space : StateSpace  A=A  B=B  C=C  D=Dd  InitialCondition=X0
  Out1 : Outport  InitialOutput=0
  wires:
  In1/1 -> State Space/1
  State Space/1 -> Out1/1

== system BenchmarkModel_Phasor/Energy Storage System2/Inverter (Phasor)/Break Alg. Loop /imag ==
  In1 : Inport
  State Space : StateSpace  A=A  B=B  C=C  D=Dd  InitialCondition=X0
  Out1 : Outport  InitialOutput=0
  wires:
  State Space/1 -> Out1/1
  In1/1 -> State Space/1

== system BenchmarkModel_Phasor/Energy Storage System2/Inverter (Phasor)/Break Alg. Loop /real ==
  In1 : Inport
  State Space : StateSpace  A=A  B=B  C=C  D=Dd  InitialCondition=X0
  Out1 : Outport  InitialOutput=0
  wires:
  State Space/1 -> Out1/1
  In1/1 -> State Space/1

== system BenchmarkModel_Phasor/Load Residential = 30 kW, PF=0.95/Residential Load1/Break Alg. Loop 1/imag1 ==
  In1 : Inport
  State Space : StateSpace  A=A  B=B  C=C  D=Dd  InitialCondition=X0
  Out1 : Outport  InitialOutput=0
  wires:
  State Space/1 -> Out1/1
  In1/1 -> State Space/1

== system BenchmarkModel_Phasor/Load Residential = 30 kW, PF=0.95/Residential Load1/Break Alg. Loop 1/real1 ==
  In1 : Inport
  State Space : StateSpace  A=A  B=B  C=C  D=Dd  InitialCondition=X0
  Out1 : Outport  InitialOutput=0
  wires:
  State Space/1 -> Out1/1
  In1/1 -> State Space/1

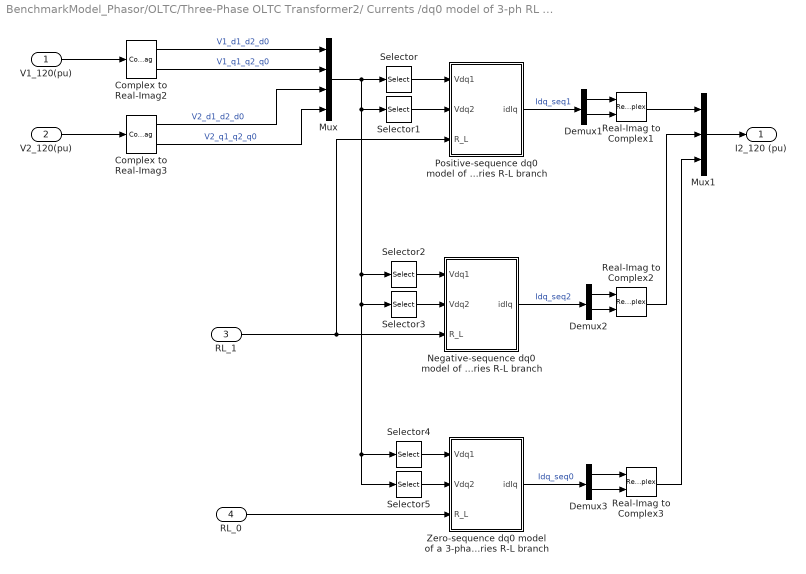
== system BenchmarkModel_Phasor/OLTC/Three-Phase OLTC Transformer2/ Currents /dq0 model of 3-ph RL branch ==
  V1_120(pu) : Inport
  V2_120(pu) : Inport  Port=2
  RL_1 : Inport  Port=3
  RL_0 : Inport  Port=4
  Complex to Real-Imag2 : ComplexToRealImag
  Complex to Real-Imag3 : ComplexToRealImag
  Demux1 : Demux  Outputs=2
      settings: DisplayOption=none
  Demux2 : Demux  Outputs=2
      settings: DisplayOption=none
  Demux3 : Demux  Outputs=2
      settings: DisplayOption=none
  Mux : Mux
  Mux1 : Mux  Inputs=3
  Negative-sequence dq0 model of a 3-phase series R-L branch : Subsystem
  Positive-sequence dq0 model of a 3-phase series R-L branch : Subsystem
  Real-Imag to Complex1 : RealImagToComplex
  Real-Imag to Complex2 : RealImagToComplex
  Real-Imag to Complex3 : RealImagToComplex
  Selector : Selector  InputPortWidth=12  IndexOptions=Index vector (dialog)  Indices=[1 4]  OutputSizes=1
  Selector1 : Selector  InputPortWidth=12  IndexOptions=Index vector (dialog)  Indices=[7 10]  OutputSizes=1
  Selector2 : Selector  InputPortWidth=12  IndexOptions=Index vector (dialog)  Indices=[1 4]+1  OutputSizes=1
  Selector3 : Selector  InputPortWidth=12  IndexOptions=Index vector (dialog)  Indices=[7 10]+1  OutputSizes=1
  Selector4 : Selector  InputPortWidth=12  IndexOptions=Index vector (dialog)  Indices=[1 4]+2  OutputSizes=1
  Selector5 : Selector  InputPortWidth=12  IndexOptions=Index vector (dialog)  Indices=[7 10]+2  OutputSizes=1
  Zero-sequence dq0 model of a 3-phase series R-L branch : Subsystem
  I2_120 (pu) : Outport
  wires:
  Positive-sequence dq0 model of a 3-phase series R-L branch/1(idIq) -> Demux1/1  "Idq_seq1"
  V1_120(pu)/1 -> Complex to Real-Imag2/1
  V2_120(pu)/1 -> Complex to Real-Imag3/1
  Selector/1 -> Positive-sequence dq0 model of a 3-phase series R-L branch/1(Vdq1)
  Selector1/1 -> Positive-sequence dq0 model of a 3-phase series R-L branch/2(Vdq2)
  Mux/1 -> Selector/1, Selector1/1, Selector2/1, Selector3/1, Selector4/1, Selector5/1
  Selector2/1 -> Negative-sequence dq0 model of a 3-phase series R-L branch/1(Vdq1)
  Selector3/1 -> Negative-sequence dq0 model of a 3-phase series R-L branch/2(Vdq2)
  Selector4/1 -> Zero-sequence dq0 model of a 3-phase series R-L branch/1(Vdq1)
  Negative-sequence dq0 model of a 3-phase series R-L branch/1(idIq) -> Demux2/1  "Idq_seq2"
  Zero-sequence dq0 model of a 3-phase series R-L branch/1(idIq) -> Demux3/1  "Idq_seq0"
  Complex to Real-Imag2/1 -> Mux/1  "V1_d1_d2_d0"
  Complex to Real-Imag2/2 -> Mux/2  "V1_q1_q2_q0"
  Complex to Real-Imag3/1 -> Mux/3  "V2_d1_d2_d0"
  Complex to Real-Imag3/2 -> Mux/4  "V2_q1_q2_q0"
  RL_1/1 -> Positive-sequence dq0 model of a 3-phase series R-L branch/3(R_L), Negative-sequence dq0 model of a 3-phase series R-L branch/3(R_L)
  Selector5/1 -> Zero-sequence dq0 model of a 3-phase series R-L branch/2(Vdq2)
  RL_0/1 -> Zero-sequence dq0 model of a 3-phase series R-L branch/3(R_L)
  Demux1/2 -> Real-Imag to Complex1/2
  Demux1/1 -> Real-Imag to Complex1/1
  Real-Imag to Complex1/1 -> Mux1/1
  Demux2/2 -> Real-Imag to Complex2/2
  Demux2/1 -> Real-Imag to Complex2/1
  Real-Imag to Complex2/1 -> Mux1/2
  Demux3/2 -> Real-Imag to Complex3/2
  Demux3/1 -> Real-Imag to Complex3/1
  Real-Imag to Complex3/1 -> Mux1/3
  Mux1/1 -> I2_120 (pu)/1

== system BenchmarkModel_Phasor/OLTC/Three-Phase OLTC Transformer2/Tap Changer Control/Determine tap position ==
  NewTap : Inport
  Trigger : TriggerPort  VariantControl=Variant
  Memory : Memory  InitialCondition=InitialPosition  InheritSampleTime=on
  Saturation : Saturate  UpperLimit=MinMaxTap(2)  LowerLimit=MinMaxTap(1)
  Sum : Sum  Inputs=|++  SaturateOnIntegerOverflow=on
  TapNo : Outport  InitialOutput=InitialPosition
  wires:
  Saturation/1 -> Memory/1, TapNo/1
  Memory/1 -> Sum/2
  Sum/1 -> Saturation/1
  NewTap/1 -> Sum/1

== system BenchmarkModel_Phasor/OLTC/Three-Phase OLTC Transformer2/Tap Changer Control/Edge Detector ==
  note: Edge or Slope Detector
  In : Inport
  Constant1 : Constant  Value=model
  Demux : Demux  Outputs=2
      settings: DisplayOption=none
  Logical Operator1 : Logic  Operator=OR
  Memory : Memory  InitialCondition=ic  LinearizeAsDelay=on
  Multiport Switch : MultiPortSwitch  SaturateOnIntegerOverflow=on
  NEGATIVE Edge : Subsystem  TreatAsAtomicUnit=on
  POSITIVE Edge : Subsystem  TreatAsAtomicUnit=on
  either edge : Constant  Value=[1 1]
  neg. edge : Constant  Value=[0 1]
  pos. edge : Constant  Value=[1 0]
  Out : Outport
  wires:
  Logical Operator1/1 -> Out/1
  NEGATIVE Edge/1(OUT) -> Logical Operator1/2
  POSITIVE Edge/1(OUT) -> Logical Operator1/1
  Memory/1 -> POSITIVE Edge/2(IN previous), NEGATIVE Edge/2(IN previous)
  In/1 -> POSITIVE Edge/1(IN), NEGATIVE Edge/1(IN), Memory/1
  pos. edge/1 -> Multiport Switch/2
  neg. edge/1 -> Multiport Switch/3
  Constant1/1 -> Multiport Switch/1
  Multiport Switch/1 -> Demux/1
  Demux/1 -> POSITIVE Edge/Enable
  Demux/2 -> NEGATIVE Edge/Enable
  either edge/1 -> Multiport Switch/4

== system BenchmarkModel_Phasor/OLTC/Three-Phase OLTC Transformer2/Z & Voltage Ratio/1st-Order Filter4 ==
  In : Inport
  State-Space : StateSpace  A=Ac  B=Bc  C=Cc  D=Dc  InitialCondition=x0c
  Out : Outport  InitialOutput=0
  wires:
  In/1 -> State-Space/1
  State-Space/1 -> Out/1
